simulink model "Q1sim5"  (R2022a)
settings: Solver=VariableStepAuto  StartTime=0.0  StopTime=9  RelTol=1e-3
values from neighbouring files (symbols this model uses):
  A = [0 0 1; 0 0 0; 92.8581 0 0]    [Q1C.m]    (also in Q1Gustavo.m = double(subs(jacobian(f),[x1 x2],[0 0])))
  B = [0; 1; -79.361]    [Q1C.m]    (also in Q1Gustavo.m = double(subs(u,[x1 x2],[0 0])))
  C = [1 0 0]    [Q1C.m]    (also in Q1Gustavo.m)
  K = lqr(A,B,Q,R)    [Q1C.m]
  L = lqr(A',C',Ql,Rl)'    [Q1C.m]
undefined symbols (not defined in the file or in its folder): x0obs
settings Model: Creator=gusta  LastModifiedBy=Crippa
settings SolverCC: ZeroCrossControl=DisableAll

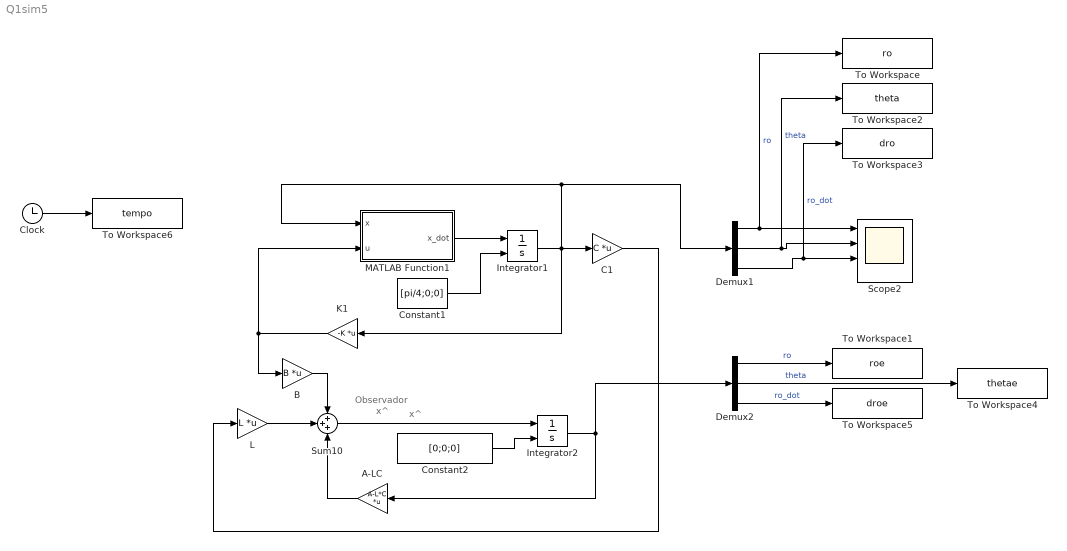
== system Q1sim5 ==
  note: Observador
  note: x^
  note: x^
  A-LC : Gain  Gain=A-L*C  Multiplication=Matrix(K*u)
  B : Gain  Gain=B  Multiplication=Matrix(K*u)
  C1 : Gain  Gain=C  Multiplication=Matrix(K*u)
  Clock : Clock
  Constant1 : Constant  Value=[pi/4;0;0]  VectorParams1D=off
  Constant2 : Constant  Value=[0;0;0]  VectorParams1D=off
  Demux1 : Demux  Outputs=3
  Demux2 : Demux  Outputs=3
  Integrator1 : Integrator  InitialConditionSource=external
  Integrator2 : Integrator  InitialConditionSource=external  InitialCondition=x0obs
  K1 : Gain  Gain=-K  Multiplication=Matrix(K*u)
  L : Gain  Gain=L  Multiplication=Matrix(K*u)
  MATLAB Function1 : MATLAB Function  TreatAsAtomicUnit=on
  Scope2 : Scope  NumInputPorts=4
  Sum10 : Sum  Inputs=+++
  To Workspace : ToWorkspace  VariableName=ro  SampleTime=-1
  To Workspace1 : ToWorkspace  VariableName=roe  SampleTime=-1
  To Workspace2 : ToWorkspace  VariableName=theta  SampleTime=-1
  To Workspace3 : ToWorkspace  VariableName=dro  SampleTime=-1
  To Workspace4 : ToWorkspace  VariableName=thetae  SampleTime=-1
  To Workspace5 : ToWorkspace  VariableName=droe  SampleTime=-1
  To Workspace6 : ToWorkspace  VariableName=tempo  SampleTime=-1
  wires:
  Integrator1/1 -> K1/1, Demux1/1, MATLAB Function1/1(x), C1/1
  Demux1/2 -> To Workspace2/1, Scope2/2  "theta"
  MATLAB Function1/1(x_dot) -> Integrator1/1
  Demux1/3 -> To Workspace3/1, Scope2/3  "ro_dot"
  Constant1/1 -> Integrator1/2
  Demux1/1 -> To Workspace/1, Scope2/1  "ro"
  C1/1 -> L/1
  Constant2/1 -> Integrator2/2
  L/1 -> Sum10/2
  B/1 -> Sum10/1
  Integrator2/1 -> Demux2/1, A-LC/1
  Sum10/1 -> Integrator2/1
  A-LC/1 -> Sum10/3
  K1/1 -> MATLAB Function1/2(u), B/1
  Demux2/1 -> To Workspace1/1  "ro"
  Demux2/2 -> To Workspace4/1  "theta"
  Demux2/3 -> To Workspace5/1  "ro_dot"
  Clock/1 -> To Workspace6/1

== matlab function Q1sim5/MATLAB Function1 ==
  data: x input; u input; x_dot output
function x_dot = gyro_model(x,u)
    %x1 = ro; x2=theta; x3=ro_dot; u=theta_dot;

    mV = .430; % [kg] massa do veículo, excluindo giroscópio e objeto
    mG = .190; % [kg] massa do giroscópio
    rG = 2*.05; % [m] raio do giroscópio
    aG = -1*.02; % [m] distância entre o centro de massa do giroscópio e ponto de rotação
    aV = .1; % [m] altura do veículo
    lV = .035; % [m] largura do veículo
    dG = .1+.02;
    dV = .1;
    omega = 3000*10472; % rpm * conversion factor = rad/sec
    g = 9.81; % [m/s^2] aceleração da gravidade
    IG11 = (mG*(rG^2)/4) + (mG*(dG^2)/12); % IG22 = IG11
    IG33 = (mG*(rG^2))/2;
    IB11 = mV*((aV^2)+(lV^2))/12;
    
    x1 = x(1);
    x2 = x(2);
    x3 = x(3);
    
    f1 = x3;
    f2 = 0;
    f3 = ((mV*dV+mG*dG)*g*sin(x1))/((IB11+mV*(dV^2)+IG11*((cos(x2))^2))+mG*(dG^2)+IG33*((sin(x2))^2));
    g1 = 0;
    g2 = 1;
    g3 = ((-2*cos(x2)*sin(x2)*x3*(IG33-IG11)-omega*cos(x2)*IG33))/((IB11+IG11*(cos(x2)^2)+mV*(dV^2)+mG*(dG^2)));

    f = [f1;f2;f3];
    g = [g1;g2;g3];

    x_dot = f + g*u;
end
